simulink model "Power_Generator3_26SimOutALT30"  (R2019a)
settings: Solver=ode23tb  StartTime=0.0  StopTime=120  RelTol=1e-4
libraries: dspnetwork x15, simulink x9, powerlib x8, sps_avr x7, dspstat3 x2
Description:
  | Copyright 2008-2019 The MathWorks, Inc.
settings Model: FPTRunName=Active  EnablePacing=on  PacingRate=0.100000  ExtModeTrigMode=oneshot  ExtModeArmWhenConnect=off  ExtModeAutoUpdateStatusClock=off  Creator=MathWorks  LastModifiedBy=Aaron
settings SolverCC: ZeroCrossAlgorithm=Adaptive
settings DataIOCC: SaveFormat=Array  SignalLoggingSaveFormat=ModelDataLogs  ReturnWorkspaceOutputs=off  SignalLoggingName=sigsOut  OutputTimes=[0:1/20:10]
settings OptimizationCC: BlockReduction=off  BooleanDataType=off  ExpressionDepthLimit=2147483647  InitFltsAndDblsToZero=on  EfficientMapNaN2IntZero=off  LifeSpan=inf
settings DebuggingCC: UnderspecifiedInitializationDetection=Classic  MergeDetectMultiDrivingBlocksExec=none  CheckExecutionContextPreStartOutputMsg=on  CheckExecutionContextRuntimeOutputMsg=on  SignalResolutionControl=TryResolveAllWithWarning  IgnoredZcDiagnostic=none  MultiTaskDSMMsg=warning  MultiTaskCondExecSysMsg=none  SigSpecEnsureSampleTimeMsg=none  FcnCallInpInsideContextMsg=warning  UnconnectedInputMsg=none  UnconnectedOutputMsg=none  UnconnectedLineMsg=none  StateNameClashWarn=warning  SFUnexpectedBacktrackingDiag=warning  SFNoUnconditionalDefaultTransitionDiag=warning  SFExecutionAtInitializationDiag=none  ArithmeticOperatorsInVariantConditions=warning
settings HardwareCC: ProdBitPerPointer=32  ProdBitPerSizeT=32  ProdBitPerPtrDiffT=32  ProdLargestAtomicFloat=None  ProdIntDivRoundTo=Undefined  ProdEndianess=Unspecified  ProdWordSize=32  ProdHWDeviceType=Specified  TargetUnknown=on
settings ModelReferenceCC: PropagateSignalLabelsOutOfModel=off
settings SFSimCC: SimUseLocalCustomCode=off
settings RTWCC: RTWUseLocalCustomCode=off
settings CodeAppCC: StateflowObjectComments=on
settings GRTTargetCC: TargetFcnLib=ansi_tfl_tmw.mat  TargetLangStandard=C89/C90 (ANSI)  GeneratePreprocessorConditionals=Disable all  CombineOutputUpdateFcns=off  GRTInterface=on
settings ConfigComp: CovMetricSettings=dw  CovHtmlReporting=on  CovSaveCumulativeToWorkspaceVar=on  CovSaveSingleToWorkspaceVar=on  CovExternalEMLEnable=off  CovSFcnEnable=off
settings SimscapeCC: SimscapeNormalizeSystem=off

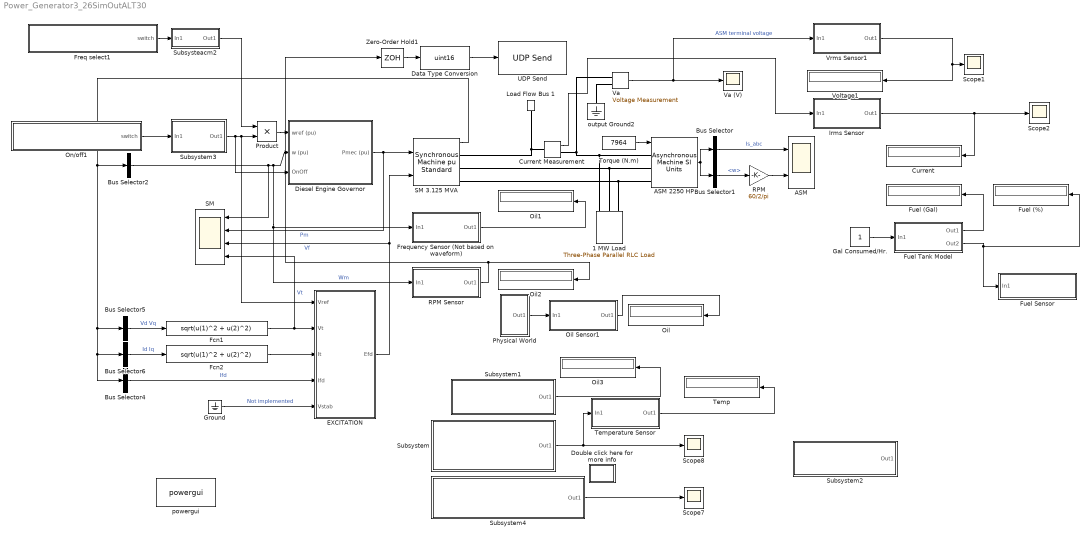
== system Power_Generator3_26SimOutALT30 ==
  1 MW Load : powerlib/Elements/Three-Phase Parallel RLC Load  LConnTagsString=A|B|C  Configuration=Y (grounded)  NominalVoltage=2400  Vabc=[1e3 1e3 1e3]  Vabcp=[1e3 1e3 1e3]  NominalFrequency=60  UnbalancedPower=off  ActivePower=1e+006  InductivePower=0  CapacitivePower=0  Pabc=[10e3 9e3 11e3]  QLabc=[100 90 110]  QCabc=[100 90 110]  Pabcp=[10e3 9e3 11e3]  QLabcp=[100 90 110]  QCabcp=[100 90 110]  Measurements=None  LoadType=constant Z
      settings: SourceProductName=Simscape Electrical
  ASM : Scope  NumInputPorts=2
  ASM 2250 HP : powerlib/Machines/Asynchronous Machine SI Units  RotorType=Squirrel-cage  PresetModel=No  MechanicalLoad=Torque Tm  ShowDetailedParameters=on  ReferenceFrame=Rotor  Units=SI  MeasurementBus=on  NominalParameters=[ 2250*746, 2400, 60 ]  Stator=[ 0.029 0.226/377]  Rotor=[ 0.022 0.226/377]  Cage1=[ 0.022 0.226/377]  Cage2=[ 0.022 0.226/377]  Lm=13.04/377  Mechanical=[ 63.87 0 2]  PolePairs=2  InitialConditions=[0 0 0 0 0 0 0 0]  SimulateSaturation=off  Saturation=[14.03593122, 27.81365428, 53.79336849, 72.68890987, 97.98006896, 148.6815601, 215.7428561, 302.9841135, 428.7778367 ; 230, 322, 414, 460, 506, 552, 598, 644, 690]  LoadFlowParameters=1492000  TsPowergui=0  TsBlock=-1  IterativeModel=Trapezoidal non iterative  IterativeDiscreteModel=Trapezoidal non iterative  Pmec=1.492e+006
      settings: SourceProductName=Simscape Electrical
  Bus Selector : BusSelector  OutputSignals=ias,ibs,ics  OutputAsBus=on
  Bus Selector1 : BusSelector  OutputSignals=w
  Bus Selector2 : BusSelector  OutputSignals="Mechanical.Rotor speed  wm  (pu)"  OutputAsBus=on
  Bus Selector4 : BusSelector  OutputSignals="dq0 components.Field current  ifd (pu)"  OutputAsBus=on
  Bus Selector5 : BusSelector  OutputSignals="dq0 components.Stator voltage  vd (pu),dq0 components.Stator voltage  vq (pu)"  OutputAsBus=on
  Bus Selector6 : BusSelector  OutputSignals="dq0 components.Stator current  id (pu),dq0 components.Stator current  iq (pu)"  OutputAsBus=on
  Current : Display
  Current Measurement : powerlib/Measurements/Current Measurement  PhasorSimulation=off  OutputType=Complex  PSBequivalent=0
      settings: SourceProductName=Simscape Electrical
  Data Type Conversion : DataTypeConversion  OutDataTypeStr=uint16
  Diesel Engine Governor : Subsystem  AncestorBlock=spsDieselMotorModel/Diesel Engine Governor  mask(Diesel Engine & Governor){K=40, Tr=[0.01 0.02 0.2], Ta=[0.25 0.009 0.0384], Tlim=[0 1.1], Td=0.024, Pm0=0}
      mask prompts: K "Regulator gain K:"; Tr "Regulator time constants [T1 T2 T3 ] (s) :"; Ta "Actuator time constants [T4 T5 T6] (s) :"; Tlim "Torque limits [Tmin Tmax] (pu) :"; Td "Engine time delay Td (s) :"; Pm0 "Initial value of mechanical power  Pm0 (pu) :"
      mask help:
      | This block implements a diesel engine and governor system. The first input is the reference speed and the second input is the measured speed. The output is the diesel engine mechanical power. The motor inertia should be combined with the generator inertia.
      |
      | The model consist of a regulator represented by the following transfer function:
      |
      |      Hc = K.(1+T3.s)/(1+T1.s+T1.T2.s^2)
      |
      | The trotte actuator is implemented as :
      |
      |      Ha =  (1+T4.s) / [ (s (1+T5.s)(1+T6.s) ]
      |
      | The motor engine is represented by a Time delay Td function.
      mask Help:
      | This block implements a diesel engine and governor system. The first input is the reference speed and the second input is the measured speed. The output is the diesel engine mechanical power. The motor inertia should be combined with the generator inertia.
      | 
      | The model consist of a regulator represented by the following transfer function:
      | 
      |      Hc = K.(1+T3.s)/(1+T1.s+T1.T2.s^2)
      | 
      | The trotte actuator is implemented as :
      | 
      |      Ha =  (1+T4.s) / [ (s (1+T5.s)(1+T6.s) ]
      | 
      | The motor engine is represented by a Time delay Td function.
  Double click here for more info : Subsystem
      settings: OpenFcn=showdemo(bdroot(gcb))
      mask Display: disp('?')
  EXCITATION : Subsystem  VariantControlMode=Label  Variant=on  LabelModeActiveChoice=Variant1
      settings: AttributesFormatString=%<BlockChoice>
  Fcn1 : Fcn  Expr=sqrt(u(1)^2 + u(2)^2)
  Fcn2 : Fcn  Expr=sqrt(u(1)^2 + u(2)^2)
  Freq select1 : Subsystem
  Frequency Sensor (Not based on waveform) : Subsystem
  Fuel (%) : Display
  Fuel (Gal) : Display
  Fuel Sensor : Subsystem
  Fuel Tank Model : Subsystem
  "Gal Consumed/Hr. " : Constant
  Ground : Ground
  Irms Sensor : Subsystem
  Load Flow Bus 1 : powerlib/Measurements/Load Flow Bus  LConnTagsString=a  Phases=single  Connectors=on one side  ID=B2  Vbase=2.4e3  Vref=1  Vangle=0  VLF=1  VLFb=1  VLFc=1  angleLF=-31.89  angleLFb=0  angleLFc=0
      settings: AttributesFormatString=%<ID>\n%<Vbase>V\n%<VLF>pu\n%<angleLF>deg.  SourceProductName=Simscape Electrical
  Oil{,1..3} (4 alike) : Display
  Oil Sensor1 : Subsystem
  On/off1 : Subsystem
  Physical World : Subsystem
  Product : Product
  RPM : Gain  Gain=60/2/pi  SaturateOnIntegerOverflow=on  OutDataTypeStr=Inherit: Same as input  ParamDataTypeStr=Inherit: Same as input
  RPM Sensor : Subsystem
  SM : Scope  NumInputPorts=4
  SM 3.125 MVA : powerlib/Machines/Synchronous Machine pu Standard  PresetModel=No  MechanicalLoad=Mechanical power Pm  ShowDetailedParameters=on  RotorType=Salient-pole  Units=per unit standard parameters  MeasurementBus=off  NominalParameters="[ 3.125e6  2400  60]"  Reactances1=[ 31 32 33 34 35 36 37 ]  Reactances2=[ 1.56, 0.296, 0.177, 1.06, 0.177, 0.052 ]  dAxisTimeConstants=Short-circuit  qAxisTimeConstants=Open-circuit  TimeConstants1=[]  TimeConstants2=[]  TimeConstants3=[]  TimeConstants4=[]  TimeConstants5=[ 3.7, 0.05, 0.05 ]  TimeConstants6=[ 8.0, 0.03, 0.3371, 0.0295 ]  TimeConstants7=[0.024 0.006 0.006]  TimeConstants8=[]  StatorResistance=0.0036  Mechanical="[ 1.07  0 2]"  PolePairs=2  InitialConditions=[0 0 0 0 0 0 0 0 1]  SetSaturation=off  Saturation=[0.211 0.418 1.0 1.25 1.72 3.35 ;0.25 0.50 1.0 1.1 1.2 1.4]  LoadFlowParameters=[1 0 0 0]  TsPowergui=0  TsBlock=-1  IterativeModel=Trapezoidal non iterative  IterativeDiscreteModel=Trapezoidal non iterative  BusType=PV  Pref=0  Qref=0  Qmin=-Inf  Qmax=Inf  PLF=0  QLF=0
      settings: AttributesFormatString=\n\n  SourceProductName=Simscape Electrical
  Scope{1..2,7..8} (4 alike) : Scope
  Subsysteacm2 : Subsystem
  Subsystem : Subsystem
  Subsystem1 : Subsystem
  Subsystem2 : Subsystem
  Subsystem3 : Subsystem
  Subsystem4 : Subsystem
  Temp : Display
  Temperature Sensor : Subsystem
  Torque (N.m) : Constant  Value=7964
  UDP Send : dspnetwork/UDP Send  remoteURL='127.0.0.1'  remotePort=25001  localURL='0.0.0.0'  localPortSource=Automatically determine  localPort=-1  sampletime=-1  blockPlatform=[]  separateLengthPort=0
      settings: SourceProductName=Simulink
  Va : powerlib/Measurements/Voltage Measurement  Tag=PoWeRsYsTeMmEaSuReMeNt  PhasorSimulation=off  OutputType=Magnitude  PSBequivalent=0
      settings: SourceProductName=Simscape Electrical
  Va (V) : Scope
  Voltage1 : Display
  Vrms Sensor1 : Subsystem
  Zero-Order Hold1 : ZeroOrderHold  SampleTime=.01
  output Ground2 : powerlib/Elements/Ground  LConnTagsString=a
      settings: SourceProductName=Simscape Electrical
  powergui : powerlib/powergui  Priority=2  SimulationMode=Discrete  SampleTime=100e-6  frequency=60  Iterations=50  frequencyindice=60  Pbase=1e6  ErrMax=0.0001  UnitsV=kV  UnitsW=MW  buscounter=0  FunctionMessages=off  echomessages=off  EnableUseOfTLC=off  CurrentSourceSwitches=off  DisableSnubberDevices=on  DisableRonSwitches=off  DisableVfSwitches=off  DisplayEquations=off  AutomaticDiscreteSolvers=off  SolverType=Tustin  Interpol=off  ExternalGateDelay=off  methode=off  Ts=0  x0status=blocks  SPID=on  SwTol=0  HookPort=off  NonlinearTolerance=0  nMaxIteration=15  ContinueOnMaxIteration=off  RestoreLinks=warning  ResistiveCurrentMeasurement=off  Frange=logspace(0,3,50)  Ylog=off  Xlog=off  ShowGrid=off  save=off  variable=ZData  structure=0  ZoomFFT=on  StartTime=0.0  cycles=2  DisplayStyle=off  fundamental=60  FreqAxis=off  MaxFrequency=1000  frequencyindicesteady=1  RmsSteady=1  display=off
      settings: SourceProductName=Simscape Electrical
  wires:
  Torque (N.m)/1 -> ASM 2250 HP/1
  ASM 2250 HP/1 -> Bus Selector/1, Bus Selector1/1
  Va/1 -> Vrms Sensor1/1(In1), Va (V)/1  "ASM terminal voltage"
  Bus Selector/1 -> ASM/1  "Is_abc"
  Bus Selector1/1 -> RPM/1  "<w>"
  RPM/1 -> ASM/2
  Diesel Engine Governor/1(Pmec (pu)) -> SM/2, SM 3.125 MVA/1  "Pm"
  Fcn2/1 -> EXCITATION/3(It)
  Bus Selector4/1 -> EXCITATION/4(Ifd)  "Ifd"
  Bus Selector6/1 -> Fcn2/1  "Id Iq"
  Ground/1 -> EXCITATION/5(Vstab)  "Not implemented"
  Bus Selector5/1 -> Fcn1/1  "Vd Vq"
  Bus Selector2/1 -> RPM Sensor/1(In1), Frequency Sensor (Not based on waveform)/1(In1), Diesel Engine Governor/2(w (pu)), SM/1  "Wm"
  Fcn1/1 -> SM/4, EXCITATION/2(Vt)  "Vt"
  EXCITATION/1(Efd) -> SM/3, SM 3.125 MVA/2  "Vf"
  SM 3.125 MVA/1 -> Bus Selector2/1, Bus Selector5/1, Bus Selector6/1, Bus Selector4/1
  Vrms Sensor1/1(Out1) -> Scope1/1, Voltage1/1
  Irms Sensor/1(Out1) -> Scope2/1, Current/1
  Current Measurement/1 -> Irms Sensor/1(In1)
  Physical World/1(Out1) -> Oil Sensor1/1(In1)
  Oil Sensor1/1(Out1) -> Oil/1
  Temperature Sensor/1(Out1) -> Temp/1
  Fuel Tank Model/1(Out1) -> Fuel (Gal)/1
  "Gal Consumed/Hr. "/1 -> Fuel Tank Model/1(In1)
  Fuel Tank Model/2(Out2) -> Fuel Sensor/1(In1), Fuel (%)/1
  Frequency Sensor (Not based on waveform)/1(Out1) -> Oil1/1
  Freq select1/1("switch ") -> Subsysteacm2/1(In1)
  On/off1/1("switch ") -> Subsystem3/1(In1)
  Product/1 -> Diesel Engine Governor/1(wref (pu))
  Subsysteacm2/1(Out1) -> Product/1
  Subsystem3/1(Out1) -> Diesel Engine Governor/3(OnOff), EXCITATION/1(Vref), Product/2
  Subsystem/1(Out1) -> Temperature Sensor/1(In1), Scope8/1
  Subsystem1/1(Out1) -> Oil3/1
  Subsystem4/1(Out1) -> Scope7/1
  Zero-Order Hold1/1 -> Data Type Conversion/1
  RPM Sensor/1(Out1) -> Zero-Order Hold1/1, Oil2/1
  Data Type Conversion/1 -> UDP Send/1
  connections:
  output Ground2/LConn1 -- Va/LConn2
  SM 3.125 MVA/RConn2 -- ASM 2250 HP/LConn2 -- 1 MW Load/LConn2
  ASM 2250 HP/LConn1 -- Current Measurement/RConn1 -- Va/LConn1 -- 1 MW Load/LConn1
  SM 3.125 MVA/RConn3 -- ASM 2250 HP/LConn3 -- 1 MW Load/LConn3
  Load Flow Bus 1/LConn1 -- SM 3.125 MVA/RConn1 -- Current Measurement/LConn1

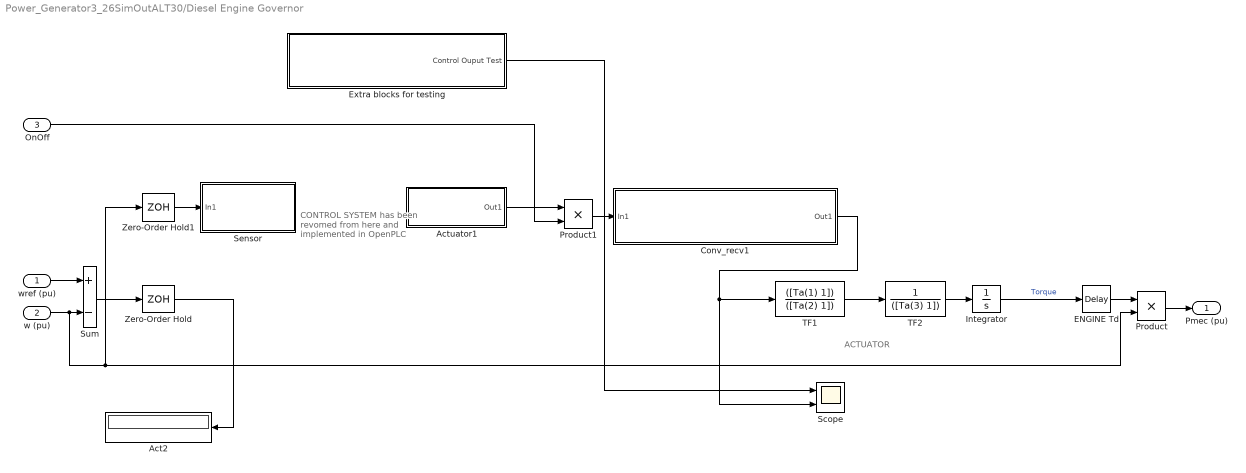
== system Power_Generator3_26SimOutALT30/Diesel Engine Governor ==
  note: ACTUATOR
  note: CONTROL SYSTEM
      | has been revomed from here
      | and implemented in
      | OpenPLC
  wref (pu) : Inport
  w (pu) : Inport  Port=2
  OnOff : Inport  Port=3
  Act2 : Display
  Actuator1 : Subsystem
  Conv_recv1 : Subsystem
  ENGINE Td : TransportDelay  DelayTime=Td  InitialOutput=Pm0
  Extra blocks for testing : Subsystem
  Integrator : Integrator  InitialCondition=Pm0  LimitOutput=on  UpperSaturationLimit=Tlim(2)  LowerSaturationLimit=Tlim(1)
  Product : Product  SaturateOnIntegerOverflow=on  InputSameDT=on  OutDataTypeStr=Inherit: Same as first input
  Product1 : Product
  Scope : Scope  NumInputPorts=2
  Sensor : Subsystem
  Sum : Sum  Inputs=+-  SaturateOnIntegerOverflow=on  InputSameDT=on  OutDataTypeStr=Inherit: Same as first input
  TF1 : TransferFcn  Numerator=([Ta(1) 1])  Denominator=([Ta(2) 1])
  TF2 : TransferFcn  Numerator=1  Denominator=([Ta(3) 1])
  Zero-Order Hold : ZeroOrderHold  SampleTime=.02
  Zero-Order Hold1 : ZeroOrderHold  SampleTime=.02
  Pmec (pu) : Outport  InitialOutput=0
  wires:
  Integrator/1 -> ENGINE Td/1  "Torque"
  TF2/1 -> Integrator/1
  Product/1 -> Pmec (pu)/1
  wref (pu)/1 -> Sum/1
  ENGINE Td/1 -> Product/1
  w (pu)/1 -> Sum/2, Zero-Order Hold1/1, Product/2
  TF1/1 -> TF2/1
  Zero-Order Hold/1 -> Act2/1
  Sum/1 -> Zero-Order Hold/1
  Conv_recv1/1(Out1) -> Scope/2, TF1/1
  Zero-Order Hold1/1 -> Sensor/1(In1)
  Extra blocks for testing/1(Control Ouput Test) -> Scope/1
  Actuator1/1(Out1) -> Product1/1
  Product1/1 -> Conv_recv1/1(In1)
  OnOff/1 -> Product1/2

== system Power_Generator3_26SimOutALT30/Double click here for more info ==

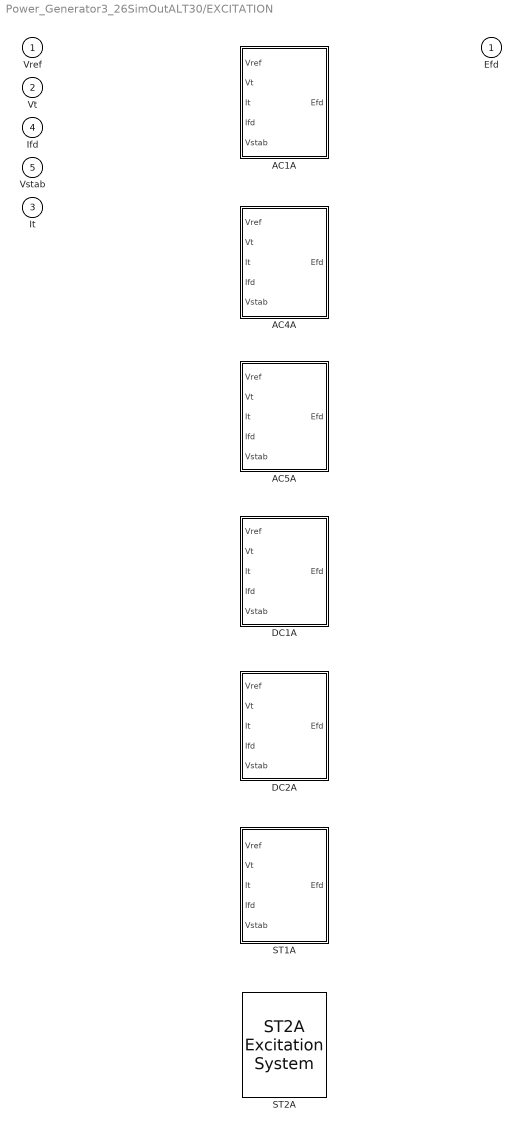
== system Power_Generator3_26SimOutALT30/EXCITATION ==
  Vref : Inport
  Vt : Inport  Port=2
  It : Inport  Port=3
  Ifd : Inport  Port=4
  Vstab : Inport  Port=5
  AC1A : Subsystem  VariantControl=Variant1
  AC4A : Subsystem  VariantControl=Variant2
  AC5A : Subsystem  VariantControl=Variant3
  DC1A : Subsystem  VariantControl=Variant4
  DC2A : Subsystem  VariantControl=Variant5
  ST1A : Subsystem  VariantControl=Variant6
  ST2A : sps_avr/ST2A Excitation System  VariantControl=Variant7  Tr=20e-3  KaTa=[120 0.15]  VRminmax=[0 1.0]  KfTf=[0.05 1.0]  KeTe=[1.0 0.5]  KI=8.0  Kp=4.88  Xd=1.56  Kc=1.82  v0=[1,1.42734]  I0=0.2739  TsBlock=-2
      settings: SourceProductName=Simscape Electrical  SourceProductBaseCode=PS
  Efd : Outport

== system Power_Generator3_26SimOutALT30/Freq select1 ==
  note: Pump Control
  Display : Display
  Terminator2 : Terminator
  UDP Receive1 : dspnetwork/UDP Receive  localURL='0.0.0.0'  localPort=20001  remoteURL='0.0.0.0'  remotePort=-1  recvBufferSize=2  dims=1  signalDatatype=int16  isComplex=off  isVarSize=off  showBlockingTime=on  blockingTime=0  sampletime=0.01  blockPlatform=LINUX
      settings: SourceProductName=DSP System Toolbox  SourceProductBaseCode=DS
  "switch " : Outport  PortDimensions=1
  wires:
  UDP Receive1/1 -> "switch "/1, Display/1
  UDP Receive1/2 -> Terminator2/1

== system Power_Generator3_26SimOutALT30/Frequency Sensor (Not based on waveform) ==
  In1 : Inport
  Downsample : DownSample  N=100  RateOptions=Allow multirate processing
  Gain : Gain  Gain=6000
  To Workspace1 : ToWorkspace  VariableName=Freq  SaveFormat=Timeseries  SampleTime=-1
  UDP Send : dspnetwork/UDP Send  remoteURL='192.168.56.106'  remotePort=10003  localURL='255.255.255.255'  localPortSource=Automatically determine  localPort=-1  sampletime=-1  blockPlatform=LINUX  separateLengthPort=0
      settings: SourceProductName=Simulink
  Zero-Order Hold : ZeroOrderHold  SampleTime=.001
  Out1 : Outport
  wires:
  In1/1 -> Zero-Order Hold/1
  Zero-Order Hold/1 -> Gain/1
  Downsample/1 -> UDP Send/1, Out1/1
  Gain/1 -> To Workspace1/1, Downsample/1

== system Power_Generator3_26SimOutALT30/Fuel Sensor ==
  In1 : Inport
  Rate Transition : RateTransition
  To Workspace1 : ToWorkspace  VariableName=Fuel  SaveFormat=Timeseries  SampleTime=-1
  UDP Send : dspnetwork/UDP Send  remoteURL='192.168.56.106'  remotePort=10005  localURL='255.255.255.255'  localPortSource=Automatically determine  localPort=-1  sampletime=-1  blockPlatform=LINUX  separateLengthPort=0
      settings: SourceProductName=Simulink
  Zero-Order Hold : ZeroOrderHold  SampleTime=.001
  Zero-Order Hold1 : ZeroOrderHold  SampleTime=0.1
  wires:
  Rate Transition/1 -> Zero-Order Hold1/1
  Zero-Order Hold1/1 -> UDP Send/1
  In1/1 -> Zero-Order Hold/1, Rate Transition/1
  Zero-Order Hold/1 -> To Workspace1/1

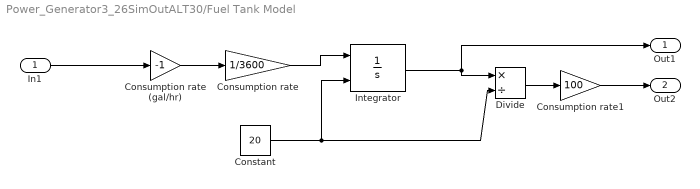
== system Power_Generator3_26SimOutALT30/Fuel Tank Model ==
  In1 : Inport
  Constant : Constant  Value=20
  Consumption rate : Gain  Gain=1/3600
  Consumption rate (gal/hr) : Gain  Gain=-1
  Consumption rate1 : Gain  Gain=100
  Divide : Product  Inputs=*/
  Integrator : Integrator  InitialConditionSource=external  InitialCondition=20  LimitOutput=on  UpperSaturationLimit=20  LowerSaturationLimit=0
  Out1 : Outport
  Out2 : Outport  Port=2
  wires:
  In1/1 -> Consumption rate (gal/hr)/1
  Constant/1 -> Divide/2, Integrator/2
  Integrator/1 -> Divide/1, Out1/1
  Consumption rate1/1 -> Out2/1
  Divide/1 -> Consumption rate1/1
  Consumption rate (gal/hr)/1 -> Consumption rate/1
  Consumption rate/1 -> Integrator/1

== system Power_Generator3_26SimOutALT30/Irms Sensor ==
  In1 : Inport
  Downsample : DownSample  N=100  RateOptions=Allow multirate processing
  RMS : dspstat3/RMS  run=on  directionMode=Entire input  dimension=1  reset_popup=None
  To Workspace1 : ToWorkspace  VariableName=Current  SaveFormat=Timeseries  SampleTime=-1
  UDP Send : dspnetwork/UDP Send  remoteURL='192.168.56.106'  remotePort=10002  localURL='255.255.255.255'  localPortSource=Automatically determine  localPort=-1  sampletime=-1  blockPlatform=LINUX  separateLengthPort=0
      settings: SourceProductName=Simulink
  Zero-Order Hold : ZeroOrderHold  SampleTime=.001
  Out1 : Outport
  wires:
  In1/1 -> Zero-Order Hold/1
  RMS/1 -> Downsample/1
  Downsample/1 -> Out1/1, UDP Send/1
  Zero-Order Hold/1 -> To Workspace1/1, RMS/1

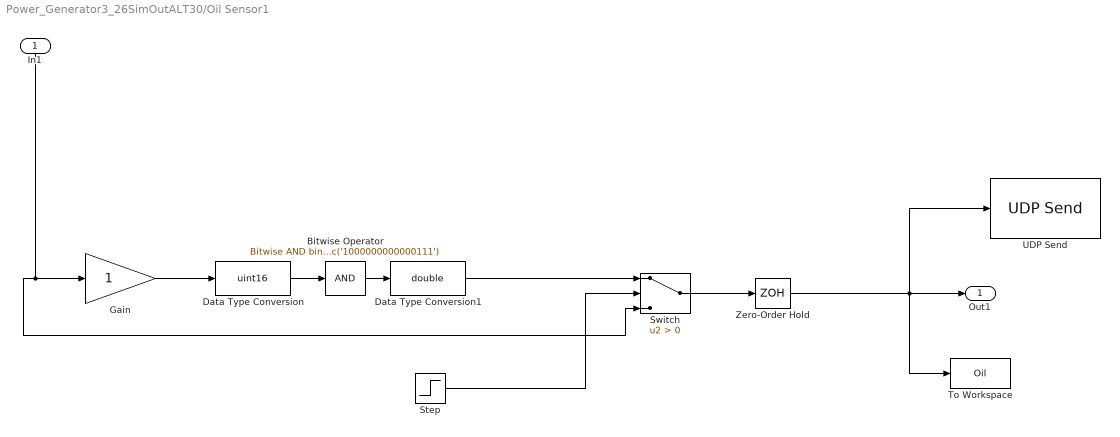
== system Power_Generator3_26SimOutALT30/Oil Sensor1 ==
  In1 : Inport
  Bitwise Operator : simulink/Logic and Bit Operations/Bitwise Operator  logicop=AND  UseBitMask=on  BitMask=bin2dec('1000000000000111')  BitMaskRealWorld=Stored Integer
  Data Type Conversion : DataTypeConversion  OutDataTypeStr=uint16
  Data Type Conversion1 : DataTypeConversion  OutDataTypeStr=double
  Gain : Gain
  Step : Step  Time=1000  SampleTime=0
  Switch : Switch  Criteria=u2 > Threshold
  To Workspace : ToWorkspace  VariableName=Oil  SaveFormat=Timeseries  SampleTime=-1
  UDP Send : dspnetwork/UDP Send  remoteURL='192.168.56.106'  remotePort=10006  localURL='255.255.255.255'  localPortSource=Automatically determine  localPort=-1  sampletime=-1  blockPlatform=LINUX  separateLengthPort=0
      settings: SourceProductName=Simulink
  Zero-Order Hold : ZeroOrderHold  SampleTime=.1
  Out1 : Outport
  wires:
  In1/1 -> Gain/1, Switch/3
  Bitwise Operator/1 -> Data Type Conversion1/1
  Gain/1 -> Data Type Conversion/1
  Data Type Conversion/1 -> Bitwise Operator/1
  Switch/1 -> Zero-Order Hold/1
  Data Type Conversion1/1 -> Switch/1
  Step/1 -> Switch/2
  Zero-Order Hold/1 -> To Workspace/1, UDP Send/1, Out1/1

== system Power_Generator3_26SimOutALT30/On//off1 ==
  note: Pump Control
  Constant : Constant  Value=0
  Display : Display
  Terminator2 : Terminator
  UDP Receive1 : dspnetwork/UDP Receive  localURL='0.0.0.0'  localPort=20002  remoteURL='0.0.0.0'  remotePort=-1  recvBufferSize=2  dims=1  signalDatatype=int16  isComplex=off  isVarSize=off  showBlockingTime=on  blockingTime=0  sampletime=0.01  blockPlatform=LINUX
      settings: SourceProductName=DSP System Toolbox  SourceProductBaseCode=DS
  "switch " : Outport  PortDimensions=1
  wires:
  UDP Receive1/2 -> Terminator2/1
  UDP Receive1/1 -> Display/1
  Constant/1 -> "switch "/1

== system Power_Generator3_26SimOutALT30/Physical World ==
  Constant2 : Constant  Value=50
  Manual Switch : ManualSwitch  CurrentSetting=0
  Step : Step  Time=.1  Before=11  After=10  SampleTime=0
  Out1 : Outport
  wires:
  Constant2/1 -> Manual Switch/1
  Step/1 -> Manual Switch/2
  Manual Switch/1 -> Out1/1

== system Power_Generator3_26SimOutALT30/RPM Sensor ==
  In1 : Inport
  Downsample : DownSample  N=100  RateOptions=Allow multirate processing
  Gain : Gain  Gain=1800
  To Workspace : ToWorkspace  VariableName=RPM  SaveFormat=Timeseries  SampleTime=-1
  UDP Send : dspnetwork/UDP Send  remoteURL='192.168.56.106'  remotePort=10004  localURL='255.255.255.255'  localPortSource=Automatically determine  localPort=-1  sampletime=-1  blockPlatform=LINUX  separateLengthPort=0
      settings: SourceProductName=Simulink
  Zero-Order Hold : ZeroOrderHold  SampleTime=.001
  Out1 : Outport
  wires:
  In1/1 -> Zero-Order Hold/1
  Zero-Order Hold/1 -> Gain/1
  Downsample/1 -> To Workspace/1, Out1/1, UDP Send/1
  Gain/1 -> Downsample/1

== system Power_Generator3_26SimOutALT30/Subsysteacm2 ==
  In1 : Inport
  Switch : Switch  Criteria=u2 > Threshold
  wref (pu) : Constant  Value=50/60
  wref (pu)1 : Constant
  Out1 : Outport
  wires:
  wref (pu)/1 -> Switch/1
  In1/1 -> Switch/2
  Switch/1 -> Out1/1
  wref (pu)1/1 -> Switch/3

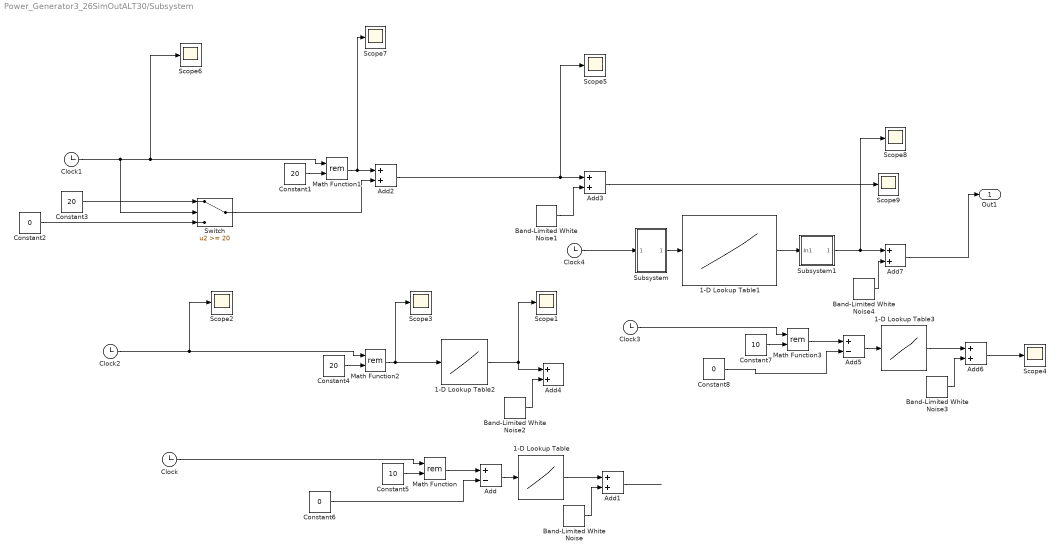
== system Power_Generator3_26SimOutALT30/Subsystem ==
  1-D Lookup Table : Lookup_n-D  NumberOfTableDimensions=1  BreakpointsForDimension1=[0 1 2 3 4 5 6 7 8 9 10]  Table=[95 160 95 110 180 110 220 150 110 220 100]  InternalRulePriority=Speed  RndMeth=Simplest  InputSameDT=on
  1-D Lookup Table1 : Lookup_n-D  NumberOfTableDimensions=1  BreakpointsForDimension1=[-0.30837,8.5726,14.922,20.379,29.22,34.058,35.577,39.571,41.237,43.63,46.905,49.828,56.556,57.797,61.814,64.292,67.193,73.554,75.769,78.17,79.044,81.033,81.979,84.656,87.149,89.905,89.987,93.175,94.549,96.778,101.24,103.47,106.65,110.57,111.14,114.63,117.6,119.98,120.13,123.16,125.7,128.88,131.01,135.5,141.14,144.45,147.56,150.59,153.73,156.99,160.98,165.73,169.45,169.5,171.18,175.91,177.62,181.59,184.09,186.45,188.61,195.56,198.78,199.61,207.62,217.68,219.2,227.71,232.61,235.43,237.48,238.93,242.15,243.14,245.15,249.13,254.02,260.34,260.79,263.14,268.75,269.26,271.33,274.56,276.67,281.73,285.92,290.5,294.12,295.39,297.31,303.34,305.85,311.88,313.56,316.73,319.6,323.15,326.7,329.11,331.23,337.12,343.52,344.26,350.01,358.75,364.6,372.85]  Table=[149.1,105.35,529.55,201.47,721.95,687.46,531.46,446.53,517.6,460.22,515.2,650.47,409.52,450.78,400.25,473.6,576.76,393.15,686.69,643.07,741.68,686.59,895.29,652.12,750.7,629.09,755.24,674.9,920.29,610.62,619.71,938.48,839.79,651.65,897.05,665.34,869.41,786.8,1023,704.17,866.97,779.75,940.26,995.23,951.55,1066.2,855.1,1155.5,1013.2,1045.3,939.71,776.78,891.39,962.49,1058.8,868.34,1005.9,875.12,985.16,872.73,1081.4,1182.2,1161.5,1186.7,1053.5,945.55,801.03,810.05,865.01,842.02,878.68,617.18,594.19,876.28,846.43,736.26,791.22,538.81,612.19,488.3,398.75,563.87,621.18,607.36,738.05,426.03,641.55,841.01,804.24,879.91,717.03,652.7,771.92,716.76,806.18,689.15,741.85,597.29,452.73,425.16,569.62,282.81,796.46,684.06,810.1,541.59,816.71,435.83]  InternalRulePriority=Speed  RndMeth=Simplest  InputSameDT=on
  1-D Lookup Table2 : Lookup_n-D  NumberOfTableDimensions=1  BreakpointsForDimension1=[0 10 20]  Table=[85 87 85]  InternalRulePriority=Speed  RndMeth=Simplest  InputSameDT=on
  1-D Lookup Table3 : Lookup_n-D  NumberOfTableDimensions=1  BreakpointsForDimension1=[0 1 2 3 4 5 6 7 8 9 10]  Table=[95 160 95 110 180 110 220 150 110 220 100]  InternalRulePriority=Speed  RndMeth=Simplest  InputSameDT=on
  Add : Sum  Inputs=+-
  Add{1..4,6..7} (6 alike) : Sum
  Add5 : Sum  Inputs=+-
  Band-Limited White Noise : simulink/Sources/Band-Limited White Noise  Cov=[0.3]  Ts=0.02  seed=[23341]
  Band-Limited White Noise1 : simulink/Sources/Band-Limited White Noise  Cov=[0.001]  Ts=0.02  seed=[233]
  Band-Limited White Noise2 : simulink/Sources/Band-Limited White Noise  Cov=[0.0001]  Ts=0.02  seed=[233]
  Band-Limited White Noise3 : simulink/Sources/Band-Limited White Noise  Cov=[0.3]  Ts=0.02  seed=[23341]
  Band-Limited White Noise4 : simulink/Sources/Band-Limited White Noise  Cov=[0.001]  Ts=0.02  seed=[233]
  Clock{,1..4} (5 alike) : Clock
  Constant1 : Constant  Value=20
  Constant2 : Constant  Value=0
  Constant3 : Constant  Value=20
  Constant4 : Constant  Value=20
  Constant5 : Constant  Value=10
  Constant6 : Constant  Value=0
  Constant7 : Constant  Value=10
  Constant8 : Constant  Value=0
  Math Function{,1..3} (4 alike) : Math  Operator=rem  SaturateOnIntegerOverflow=on
  Scope{1..9} (9 alike) : Scope
  Subsystem : Subsystem
  Subsystem1 : Subsystem
  Switch : Switch  Threshold=20
  Out1 : Outport
  wires:
  Constant3/1 -> Switch/1
  Math Function1/1 -> Scope7/1, Add2/1
  Switch/1 -> Add2/2
  Constant2/1 -> Switch/3
  Band-Limited White Noise1/1 -> Add3/2
  Add3/1 -> Scope9/1
  Constant1/1 -> Math Function1/2
  Clock1/1 -> Switch/2, Scope6/1, Math Function1/1
  Add2/1 -> Scope5/1, Add3/1
  Math Function2/1 -> Scope3/1, 1-D Lookup Table2/1
  Band-Limited White Noise2/1 -> Add4/2
  Constant4/1 -> Math Function2/2
  Clock2/1 -> Scope2/1, Math Function2/1
  1-D Lookup Table2/1 -> Add4/1, Scope1/1
  Constant5/1 -> Math Function/2
  1-D Lookup Table/1 -> Add1/1
  Add1/1 -> ?
  Clock/1 -> Math Function/1
  Add/1 -> 1-D Lookup Table/1
  Band-Limited White Noise/1 -> Add1/2
  Constant6/1 -> Add/2
  Math Function/1 -> Add/1
  Constant7/1 -> Math Function3/2
  1-D Lookup Table3/1 -> Add6/1
  Add6/1 -> Scope4/1
  Clock3/1 -> Math Function3/1
  Add5/1 -> 1-D Lookup Table3/1
  Band-Limited White Noise3/1 -> Add6/2
  Constant8/1 -> Add5/2
  Math Function3/1 -> Add5/1
  Band-Limited White Noise4/1 -> Add7/2
  Add7/1 -> Out1/1
  Clock4/1 -> Subsystem/1(In1)
  Subsystem/1(Out1) -> 1-D Lookup Table1/1
  Subsystem1/1(Out1) -> Scope8/1, Add7/1
  1-D Lookup Table1/1 -> Subsystem1/1(In1)

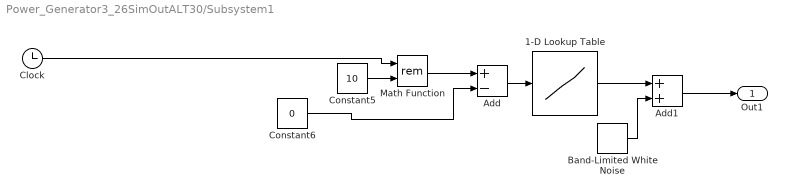
== system Power_Generator3_26SimOutALT30/Subsystem1 ==
  1-D Lookup Table : Lookup_n-D  NumberOfTableDimensions=1  BreakpointsForDimension1=[0 1 2 3 4 5 6 7 8 9 10]  Table=[95 160 95 110 180 110 220 150 110 220 100]  InternalRulePriority=Speed  RndMeth=Simplest  InputSameDT=on
  Add : Sum  Inputs=+-
  Add1 : Sum
  Band-Limited White Noise : simulink/Sources/Band-Limited White Noise  Cov=[0.3]  Ts=0.02  seed=[23341]
  Clock : Clock
  Constant5 : Constant  Value=10
  Constant6 : Constant  Value=0
  Math Function : Math  Operator=rem  SaturateOnIntegerOverflow=on
  Out1 : Outport
  wires:
  Band-Limited White Noise/1 -> Add1/2
  Add/1 -> 1-D Lookup Table/1
  Constant6/1 -> Add/2
  Constant5/1 -> Math Function/2
  Math Function/1 -> Add/1
  Clock/1 -> Math Function/1
  Add1/1 -> Out1/1
  1-D Lookup Table/1 -> Add1/1

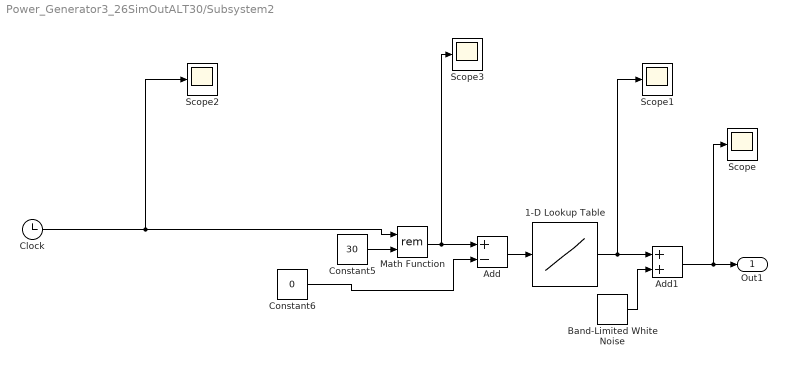
== system Power_Generator3_26SimOutALT30/Subsystem2 ==
  1-D Lookup Table : Lookup_n-D  NumberOfTableDimensions=1  BreakpointsForDimension1=[0 15 30]  Table=[84 87 84]  InternalRulePriority=Speed  RndMeth=Simplest  InputSameDT=on
  Add : Sum  Inputs=+-
  Add1 : Sum
  Band-Limited White Noise : simulink/Sources/Band-Limited White Noise  Cov=[0.3]  Ts=0.02  seed=[23341]
  Clock : Clock
  Constant5 : Constant  Value=30
  Constant6 : Constant  Value=0
  Math Function : Math  Operator=rem  SaturateOnIntegerOverflow=on
  Scope{,1..3} (4 alike) : Scope
  Out1 : Outport
  wires:
  Band-Limited White Noise/1 -> Add1/2
  Add/1 -> 1-D Lookup Table/1
  Constant6/1 -> Add/2
  Constant5/1 -> Math Function/2
  Math Function/1 -> Scope3/1, Add/1
  Add1/1 -> Scope/1, Out1/1
  1-D Lookup Table/1 -> Scope1/1, Add1/1
  Clock/1 -> Scope2/1, Math Function/1

== system Power_Generator3_26SimOutALT30/Subsystem3 ==
  In1 : Inport
  Subtract : Sum  Inputs=+-
  "Vtref (pu) " : Constant
  Out1 : Outport
  wires:
  "Vtref (pu) "/1 -> Subtract/1
  In1/1 -> Subtract/2
  Subtract/1 -> Out1/1

== system Power_Generator3_26SimOutALT30/Subsystem4 ==
  Rate Transition : RateTransition
  Step2 : Step  Time=.1  SampleTime=0
  UDP Send : dspnetwork/UDP Send  remoteURL='192.168.56.106'  remotePort=10009  localURL='255.255.255.255'  localPortSource=Automatically determine  localPort=-1  sampletime=-1  blockPlatform=LINUX  separateLengthPort=0
      settings: SourceProductName=DSP System Toolbox  SourceProductBaseCode=DS
  Zero-Order Hold : ZeroOrderHold  SampleTime=0.05
  Out1 : Outport
  wires:
  Rate Transition/1 -> Zero-Order Hold/1
  Zero-Order Hold/1 -> Out1/1, UDP Send/1
  Step2/1 -> Rate Transition/1

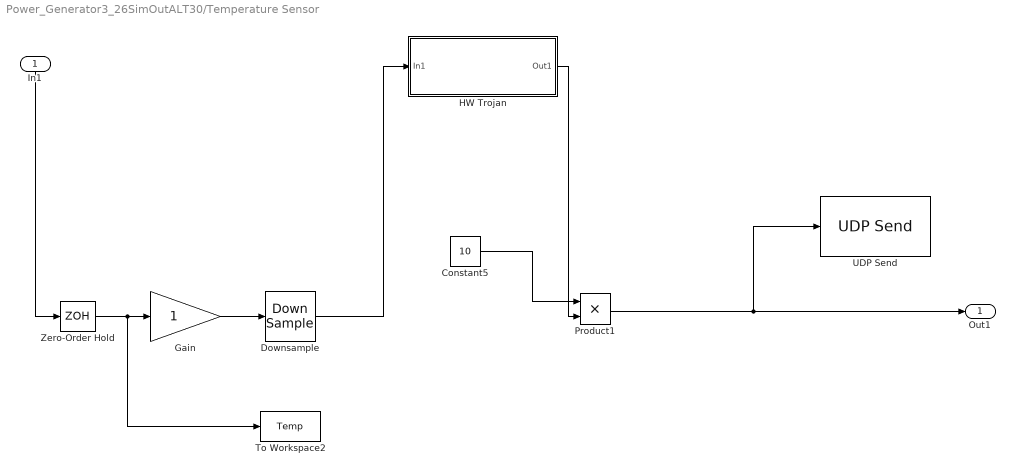
== system Power_Generator3_26SimOutALT30/Temperature Sensor ==
  In1 : Inport
  Constant5 : Constant  Value=10
  Downsample : DownSample  N=100  RateOptions=Allow multirate processing
  Gain : Gain
  HW Trojan : Subsystem
  Product1 : Product
  To Workspace2 : ToWorkspace  VariableName=Temp  SaveFormat=Timeseries  SampleTime=-1
  UDP Send : dspnetwork/UDP Send  remoteURL='192.168.56.106'  remotePort=10007  localURL='255.255.255.255'  localPortSource=Automatically determine  localPort=-1  sampletime=-1  blockPlatform=LINUX  separateLengthPort=0
      settings: SourceProductName=Simulink
  Zero-Order Hold : ZeroOrderHold  SampleTime=.001
  Out1 : Outport
  wires:
  In1/1 -> Zero-Order Hold/1
  Gain/1 -> Downsample/1
  Zero-Order Hold/1 -> To Workspace2/1, Gain/1
  Downsample/1 -> HW Trojan/1(In1)
  Constant5/1 -> Product1/1
  Product1/1 -> UDP Send/1, Out1/1
  HW Trojan/1(Out1) -> Product1/2

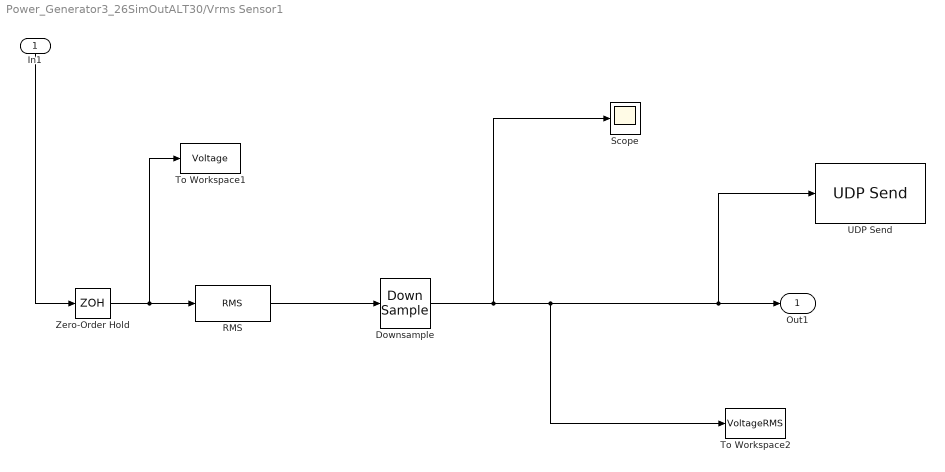
== system Power_Generator3_26SimOutALT30/Vrms Sensor1 ==
  In1 : Inport
  Downsample : DownSample  N=100  RateOptions=Allow multirate processing
  RMS : dspstat3/RMS  run=on  directionMode=Entire input  dimension=1  reset_popup=None
  Scope : Scope
  To Workspace1 : ToWorkspace  VariableName=Voltage  SaveFormat=Timeseries  SampleTime=-1
  To Workspace2 : ToWorkspace  VariableName=VoltageRMS  SaveFormat=Timeseries  SampleTime=-1
  UDP Send : dspnetwork/UDP Send  remoteURL='192.168.56.106'  remotePort=10001  localURL='255.255.255.255'  localPortSource=Automatically determine  localPort=-1  sampletime=-1  blockPlatform=LINUX  separateLengthPort=0
      settings: SourceProductName=Simulink
  Zero-Order Hold : ZeroOrderHold  SampleTime=.001
  Out1 : Outport
  wires:
  In1/1 -> Zero-Order Hold/1
  RMS/1 -> Downsample/1
  Zero-Order Hold/1 -> To Workspace1/1, RMS/1
  Downsample/1 -> Scope/1, To Workspace2/1, Out1/1, UDP Send/1

== system Power_Generator3_26SimOutALT30/Diesel Engine Governor/Actuator1 ==
  UDP Receive : dspnetwork/UDP Receive  localURL='0.0.0.0'  localPort=40002  remoteURL='0.0.0.0'  remotePort=-1  recvBufferSize=2  dims=1  signalDatatype=uint16  isComplex=off  isVarSize=off  showBlockingTime=on  blockingTime=0  sampletime=-1  blockPlatform=LINUX
      settings: SourceProductName=Simulink
  Voltage1 : Display
  Voltage2 : Display
  Out1 : Outport
  wires:
  UDP Receive/1 -> Out1/1, Voltage1/1
  UDP Receive/2 -> Voltage2/1

== system Power_Generator3_26SimOutALT30/Diesel Engine Governor/Conv_recv1 ==
  In1 : Inport
  Constant : Constant  Value=10000
  Constant1 : Constant  Value=10000
  Divide : Product  Inputs=*/
  Sum2 : Sum  Inputs=|+-
  Out1 : Outport
  wires:
  In1/1 -> Sum2/1
  Divide/1 -> Out1/1
  Sum2/1 -> Divide/1
  Constant/1 -> Sum2/2
  Constant1/1 -> Divide/2

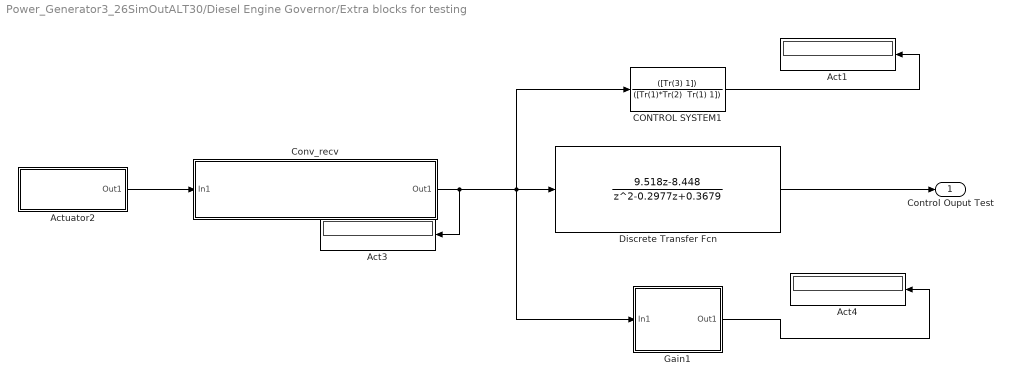
== system Power_Generator3_26SimOutALT30/Diesel Engine Governor/Extra blocks for testing ==
  Act1 : Display
  Act3 : Display
  Act4 : Display
  Actuator2 : Subsystem
  CONTROL SYSTEM1 : TransferFcn  Numerator=([Tr(3) 1])  Denominator="([Tr(1)*Tr(2)  Tr(1) 1])"
  Conv_recv : Subsystem
  Discrete Transfer Fcn : DiscreteTransferFcn  Numerator=[9.518 -8.448]  Denominator=[1 -0.2977 0.3679]  SampleTime=.02
  Gain1 : Subsystem
  Control Ouput Test : Outport  InitialOutput=0
  wires:
  Actuator2/1(Out1) -> Conv_recv/1(In1)
  Conv_recv/1(Out1) -> Act3/1, Gain1/1(In1), CONTROL SYSTEM1/1, Discrete Transfer Fcn/1
  CONTROL SYSTEM1/1 -> Act1/1
  Gain1/1(Out1) -> Act4/1
  Discrete Transfer Fcn/1 -> Control Ouput Test/1

== system Power_Generator3_26SimOutALT30/Diesel Engine Governor/Sensor ==
  In1 : Inport
  Conv_send : Subsystem
  Sensor : Subsystem
  wires:
  In1/1 -> Conv_send/1(In1)
  Conv_send/1(Out1) -> Sensor/1(In1)

== system Power_Generator3_26SimOutALT30/EXCITATION/AC1A ==
  Vref : Inport
  Vt : Inport  Port=2
  It : Inport  Port=3
  Ifd : Inport  Port=4
  Vstab : Inport  Port=5
  AC1A : sps_avr/AC1A Excitation System  Tr=20e-3  KaTa=[400 0.02]  VAminmax=[-14.5 14.5]  VRminmax=[-5.43 6.03]  KfTf=[0.03 1.0]  TbTc=[0 0]  KeTe=[1.0 0.80]  Ve12=[4.18 3.14]  SeVe12=[0.10 0.03]  Kd=0.38  Kc=0.20  v0=[1 1.4273]  TsBlock=-2
      settings: SourceProductName=Simscape Electrical  SourceProductBaseCode=PS
  term3 : Terminator
  Efd : Outport
  wires:
  It/1 -> term3/1
  AC1A/1 -> Efd/1
  Vstab/1 -> AC1A/4
  Ifd/1 -> AC1A/3
  Vt/1 -> AC1A/2
  Vref/1 -> AC1A/1

== system Power_Generator3_26SimOutALT30/EXCITATION/AC4A ==
  Vref : Inport
  Vt : Inport  Port=2
  It : Inport  Port=3
  Ifd : Inport  Port=4
  Vstab : Inport  Port=5
  AC4A : sps_avr/AC4A Excitation System  Tr=20e-3  KaTa=[200 0.015]  VIminmax=[-10 10]  VRminmax=[-4.53 5.64]  TbTc=[10 1.0]  Kc=0  v0=[1,1.42734]  TsBlock=-2
      settings: SourceProductName=Simscape Electrical  SourceProductBaseCode=PS
  term3 : Terminator
  Efd : Outport
  wires:
  It/1 -> term3/1
  AC4A/1 -> Efd/1
  Vstab/1 -> AC4A/4
  Ifd/1 -> AC4A/3
  Vt/1 -> AC4A/2
  Vref/1 -> AC4A/1

== system Power_Generator3_26SimOutALT30/EXCITATION/AC5A ==
  Vref : Inport
  Vt : Inport  Port=2
  It : Inport  Port=3
  Ifd : Inport  Port=4
  Vstab : Inport  Port=5
  AC5A : sps_avr/AC5A Excitation System  Tr=20e-3  KaTa=[100 0.02]  VRminmax=[-7.3 7.3]  KfTf=[0.03 1 0 0]  KeTe=[1.0 0.02]  Efd12=[5.6 0.75*5.6]  SeEfd12=[0.86 0.5]  v0=[1,1.42734]  TsBlock=-2
      settings: SourceProductName=Simscape Electrical  SourceProductBaseCode=PS
  term3 : Terminator
  term4 : Terminator
  Efd : Outport
  wires:
  Ifd/1 -> term4/1
  It/1 -> term3/1
  AC5A/1 -> Efd/1
  Vstab/1 -> AC5A/3
  Vt/1 -> AC5A/2
  Vref/1 -> AC5A/1

== system Power_Generator3_26SimOutALT30/EXCITATION/DC1A ==
  Vref : Inport
  Vt : Inport  Port=2
  It : Inport  Port=3
  Ifd : Inport  Port=4
  Vstab : Inport  Port=5
  DC1A : sps_avr/DC1A Excitation System  Tr=20e-3  KaTa=[46 0.06]  VRminmax=[-0.9 1.0]  KfTf=[0.05 1.5]  TbTc=[0 0]  KeTe=[0.05 0.46]  Efd12=[3.1 2.3]  SeEfd12=[0.33 0.10]  v0=[1,1.42734]  TsBlock=-2
      settings: SourceProductName=Simscape Electrical  SourceProductBaseCode=PS
  term3 : Terminator
  term4 : Terminator
  Efd : Outport
  wires:
  Ifd/1 -> term4/1
  It/1 -> term3/1
  DC1A/1 -> Efd/1
  Vstab/1 -> DC1A/3
  Vt/1 -> DC1A/2
  Vref/1 -> DC1A/1

== system Power_Generator3_26SimOutALT30/EXCITATION/DC2A ==
  Vref : Inport
  Vt : Inport  Port=2
  It : Inport  Port=3
  Ifd : Inport  Port=4
  Vstab : Inport  Port=5
  DC2A : sps_avr/DC2A Excitation System  Tr=20e-3  KaTa=[46 0.06]  VRminmax=[-4.9 4.95]  KfTf=[0.05 1.5]  TbTc=[0 0]  KeTe=[0.05 0.46]  Efd12=[3.05 2.29]  SeEfd12=[0.279 0.117]  v0=[1,1.42734]  TsBlock=-2
      settings: SourceProductName=Simscape Electrical  SourceProductBaseCode=PS
  term3 : Terminator
  term4 : Terminator
  Efd : Outport
  wires:
  Ifd/1 -> term4/1
  It/1 -> term3/1
  DC2A/1 -> Efd/1
  Vstab/1 -> DC2A/3
  Vt/1 -> DC2A/2
  Vref/1 -> DC2A/1

== system Power_Generator3_26SimOutALT30/EXCITATION/ST1A ==
  Vref : Inport
  Vt : Inport  Port=2
  It : Inport  Port=3
  Ifd : Inport  Port=4
  Vstab : Inport  Port=5
  ST1A : sps_avr/ST1A Excitation System  Tr=20e-3  KaTa=[210 0.001]  VIminmax=[-999 999]  VAminmax=[-999 999]  VRminmax=[-6.0 6.43]  KfTf=[0.001 1]  TbTc=[0 0 0 0]  KLR=1  ILR=2  Kc=0.038  v0=[1,1.42734]  TsBlock=-2
      settings: SourceProductName=Simscape Electrical  SourceProductBaseCode=PS
  term3 : Terminator
  Efd : Outport
  wires:
  It/1 -> term3/1
  ST1A/1 -> Efd/1
  Vstab/1 -> ST1A/4
  Ifd/1 -> ST1A/3
  Vt/1 -> ST1A/2
  Vref/1 -> ST1A/1

== system Power_Generator3_26SimOutALT30/Subsystem/Subsystem ==
  In1 : Inport
  Constant : Constant  Value=.25
  Product : Product
  Out1 : Outport
  wires:
  Constant/1 -> Product/2
  In1/1 -> Product/1
  Product/1 -> Out1/1

== system Power_Generator3_26SimOutALT30/Subsystem/Subsystem1 ==
  In1 : Inport
  Constant9 : Constant  Value=3
  Divide : Product  Inputs=*/
  Out1 : Outport
  wires:
  Constant9/1 -> Divide/2
  In1/1 -> Divide/1
  Divide/1 -> Out1/1

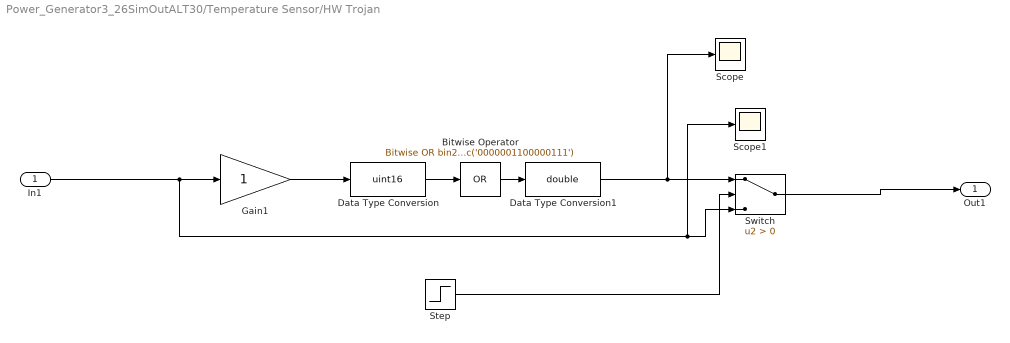
== system Power_Generator3_26SimOutALT30/Temperature Sensor/HW Trojan ==
  In1 : Inport
  Bitwise Operator : simulink/Logic and Bit Operations/Bitwise Operator  logicop=OR  UseBitMask=on  BitMask=bin2dec('0000001100000111')  BitMaskRealWorld=Stored Integer
  Data Type Conversion : DataTypeConversion  OutDataTypeStr=uint16
  Data Type Conversion1 : DataTypeConversion  OutDataTypeStr=double
  Gain1 : Gain
  Scope : Scope
  Scope1 : Scope
  Step : Step  Time=50  SampleTime=0
  Switch : Switch  Criteria=u2 > Threshold
  Out1 : Outport
  wires:
  In1/1 -> Scope1/1, Switch/3, Gain1/1
  Data Type Conversion1/1 -> Scope/1, Switch/1
  Bitwise Operator/1 -> Data Type Conversion1/1
  Gain1/1 -> Data Type Conversion/1
  Step/1 -> Switch/2
  Data Type Conversion/1 -> Bitwise Operator/1
  Switch/1 -> Out1/1

== system Power_Generator3_26SimOutALT30/Diesel Engine Governor/Extra blocks for testing/Actuator2 ==
  To Workspace : ToWorkspace  VariableName=Act  SaveFormat=Timeseries  SampleTime=-1
  UDP Receive : dspnetwork/UDP Receive  localURL='0.0.0.0'  localPort=40001  remoteURL='0.0.0.0'  remotePort=-1  recvBufferSize=2  dims=1  signalDatatype=uint16  isComplex=off  isVarSize=off  showBlockingTime=on  blockingTime=0  sampletime=-1  blockPlatform=LINUX
      settings: SourceProductName=Simulink
  Voltage1 : Display
  Voltage2 : Display
  Out1 : Outport
  wires:
  UDP Receive/2 -> Voltage2/1
  UDP Receive/1 -> Voltage1/1, Out1/1, To Workspace/1

== system Power_Generator3_26SimOutALT30/Diesel Engine Governor/Extra blocks for testing/Conv_recv ==
  In1 : Inport
  Constant : Constant  Value=10000
  Constant1 : Constant  Value=10000
  Divide : Product  Inputs=*/
  Sum2 : Sum  Inputs=|+-
  Out1 : Outport
  wires:
  In1/1 -> Sum2/1
  Divide/1 -> Out1/1
  Sum2/1 -> Divide/1
  Constant/1 -> Sum2/2
  Constant1/1 -> Divide/2

== system Power_Generator3_26SimOutALT30/Diesel Engine Governor/Extra blocks for testing/Gain1 ==
  In1 : Inport
  Custom Gain Actuator : Subsystem
  Gain K : Gain  Gain=-1  SaturateOnIntegerOverflow=on  OutDataTypeStr=Inherit: Same as input  ParamDataTypeStr=Inherit: Same as input
  Product1 : Product
  Out1 : Outport
  wires:
  Gain K/1 -> Product1/1
  Product1/1 -> Out1/1
  Custom Gain Actuator/1(Out1) -> Product1/2
  In1/1 -> Gain K/1

== system Power_Generator3_26SimOutALT30/Diesel Engine Governor/Sensor/Conv_send ==
  In1 : Inport
  Constant : Constant  Value=10000
  Constant1 : Constant  Value=10000
  Product1 : Product
  Sum1 : Sum  Inputs=|++
  Out1 : Outport
  wires:
  Product1/1 -> Sum1/1
  In1/1 -> Product1/1
  Sum1/1 -> Out1/1
  Constant1/1 -> Sum1/2
  Constant/1 -> Product1/2

== system Power_Generator3_26SimOutALT30/Diesel Engine Governor/Sensor/Sensor ==
  In1 : Inport
  Scope : Scope
  To Workspace : ToWorkspace  VariableName=sen  SaveFormat=Timeseries  SampleTime=-1
  UDP Send : dspnetwork/UDP Send  remoteURL='192.168.56.106'  remotePort=10008  localURL='255.255.255.255'  localPortSource=Automatically determine  localPort=-1  sampletime=-1  blockPlatform=LINUX  separateLengthPort=0
      settings: SourceProductName=Simulink
  Zero-Order Hold : ZeroOrderHold  SampleTime=.01
  wires:
  In1/1 -> Zero-Order Hold/1
  Zero-Order Hold/1 -> Scope/1, To Workspace/1, UDP Send/1

== system Power_Generator3_26SimOutALT30/Diesel Engine Governor/Extra blocks for testing/Gain1/Custom Gain Actuator ==
  Constant : Constant
  UDP Receive1 : dspnetwork/UDP Receive  localURL='0.0.0.0'  localPort=40002  remoteURL='0.0.0.0'  remotePort=-1  recvBufferSize=8192  dims=1  signalDatatype=uint16  isComplex=off  isVarSize=off  showBlockingTime=on  blockingTime=0  sampletime=0.01  blockPlatform=LINUX
      settings: SourceProductName=Simulink
  Voltage1 : Display
  Voltage2 : Display
  Out1 : Outport
  wires:
  Constant/1 -> Out1/1
  UDP Receive1/1 -> Voltage1/1
  UDP Receive1/2 -> Voltage2/1
